simulink model "simulazione_sistema_con_errore"  (R2019b)
settings: Solver=VariableStepAuto  StartTime=0.0  StopTime=50  RelTol=1e-3
values from neighbouring files (symbols this model uses):
  A = [0 0 1 0;0 0 0 1;-k/m1 k/m1 -c/m1 c/m1;k/m2 -k/m2 c/m2 -c/m2]    [ValoriCaso1.m]    (also in ValoriCaso2.m; ValoriCaso3.m; ValoriCaso4.m; ValoriCaso5.m)
  B = [0;0;1/m1;0]    [ValoriCaso1.m]    (also in ValoriCaso2.m; ValoriCaso3.m; ValoriCaso4.m; ValoriCaso5.m)
  C = [1 0 0 0]    [ValoriCaso1.m]    (also in ValoriCaso2.m; ValoriCaso3.m; ValoriCaso4.m; ValoriCaso5.m)
  V = -(Fd')    [CreazioneOsservatore.m]
undefined symbols (not defined in the file or in its folder): mat_f
settings Model: Creator=sugam  LastModifiedBy=sugam

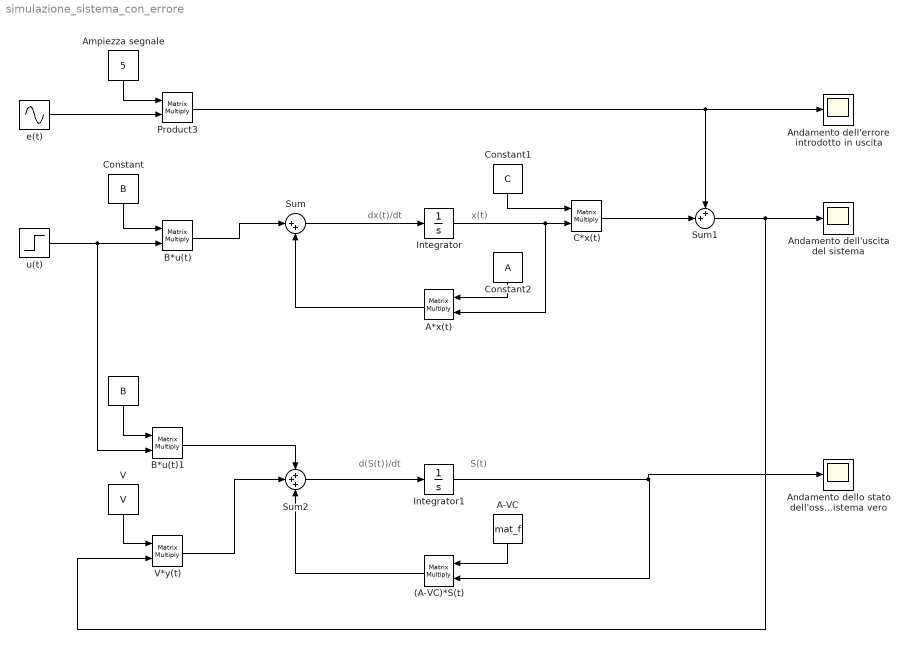
== system simulazione_sistema_con_errore ==
  note: x(t)
  note: dx(t)/dt
  note: S(t)
  note: d(S(t))/dt
  " " : Constant  Value=B  SampleTime=0
  (A-VC)*S(t) : Product  Multiplication=Matrix(*)
  A*x(t) : Product  Multiplication=Matrix(*)
  A-VC : Constant  Value=mat_f  VectorParams1D=off  SampleTime=0
  Ampiezza segnale : Constant  Value=5  VectorParams1D=off  SampleTime=0
  Andamento dell'errore introdotto in uscita : Scope
  Andamento dell'uscita del sistema : Scope
  Andamento dello stato dell'osservatore che simula quello del sistema vero : Scope
  B*u(t) : Product  Multiplication=Matrix(*)
  B*u(t)1 : Product  Multiplication=Matrix(*)
  C*x(t) : Product  Multiplication=Matrix(*)
  Constant : Constant  Value=B  VectorParams1D=off
  Constant1 : Constant  Value=C  VectorParams1D=off
  Constant2 : Constant  Value=A  VectorParams1D=off
  Integrator : Integrator
  Integrator1 : Integrator
  Product3 : Product  Multiplication=Matrix(*)
  Sum : Sum  Inputs=|++
  Sum1 : Sum  Inputs=++|
  Sum2 : Sum  Inputs=+++
  V : Constant  Value=V  VectorParams1D=off  SampleTime=0
  V*y(t) : Product  Multiplication=Matrix(*)
  e(t) : Sin  Frequency=5  SampleTime=0
  u(t) : Step  Time=5  SampleTime=0
  wires:
  u(t)/1 -> B*u(t)1/2, B*u(t)/2
  Constant/1 -> B*u(t)/1
  B*u(t)/1 -> Sum/1
  Sum/1 -> Integrator/1
  Integrator/1 -> A*x(t)/2, C*x(t)/2
  Constant1/1 -> C*x(t)/1
  Constant2/1 -> A*x(t)/1
  A*x(t)/1 -> Sum/2
  Ampiezza segnale/1 -> Product3/1
  e(t)/1 -> Product3/2
  Product3/1 -> Andamento dell'errore introdotto in uscita/1, Sum1/1
  C*x(t)/1 -> Sum1/2
  Sum1/1 -> V*y(t)/2, Andamento dell'uscita del sistema/1
  (A-VC)*S(t)/1 -> Sum2/3
  Integrator1/1 -> Andamento dello stato dell'osservatore che simula quello del sistema vero/1, (A-VC)*S(t)/2
  V/1 -> V*y(t)/1
  A-VC/1 -> (A-VC)*S(t)/1
  V*y(t)/1 -> Sum2/2
  B*u(t)1/1 -> Sum2/1
  " "/1 -> B*u(t)1/1
  Sum2/1 -> Integrator1/1
